simulink model "old"  (R2022b)
settings: Solver=FixedStepAuto  StartTime=1000  StopTime=1100  FixedStep=0.01  RelTol=1e-3
model workspace (MATLAB code in the model file):
  | A = ...
  |   [1 0.02;
  |    0 1];
  | 
  | B = [0.0002; 0.02];
  | 
  | C = [0 1];
  | 
  | I = ...
  |   [1 0;
  |    0 1];
  | 
  | P0 = ...
  |   [1 0;
  |    0 1];
  | 
  | PotenciaNegativa = -50000;
  | 
  | PotenciaPositiva = 80000;
  | 
  | Q = ...
  |   [10 0;
  |    0 10];
  | 
  | R = 1000;
  | 
  | T = 0.02;
  | 
  | TorqueMaxNegative = -12;
  | 
  | TorqueMaxPositive = 21;
  | 
  | diff_table_F = [0 0.0005 0.0005 0.0006 0.0006 0.0007 0.0008 0.0008 0.0009 ...
  |                 0.0009 0.001 0.0011 0.0011 0.0012 0.0013 0.0014 0.0014 ...
  |                 0.0015 0.0016 0.0017 0.0018 0.0018 0.0019 0.002 0.0021 ...
  |                 0.0022 0.0023 0.0024 0.0025 0.0026 0.0027 0.0027 0.0028 ...
  |                 0.0029 0.0031 0.0032 0.0033 0.0034 0.0035 0.0036 0.0037 ...
  |                 0.0038 0.0039 0.004 0.0042 0.0043 0.0044 0.0045 0.0046 ...
  |                 0.0048 0.0049 0.005 0.0051 0.0053 0.0054 0.0055 0.0057 ...
  |                 0.0058 0.0059 0.0061 0.0062 0.0064 0.0065 0.0067 0.0068 ...
  |                 0.007 0.0071 0.0073 0.0074 0.0076 0.0077 0.0079 0.008 0.0082 ...
  |                 0.0084 0.0085 0.0087 0.0089 0.009 0.0092 0.0094 0.0095];
  | 
  | diff_table_R = [0 0.0023 0.00253 0.00276 0.00299 0.00322 0.00345 0.00368 ...
  |                 0.00391 0.00414 0.00437 0.0046 0.00483 0.00506 0.00529 ...
  |                 0.00552 0.00575 0.00598 0.00621 0.00644 0.00667 0.0069 ...
  |                 0.00713 0.00736 0.00759 0.00782 0.00805 0.00828 0.00851 ...
  |                 0.00874 0.00897 0.0092 0.00943 0.00966 0.00989 0.01012 ...
  |                 0.01035 0.01058 0.01081 0.01104 0.01127 0.0115 0.01173 ...
  |                 0.01196 0.01219 0.01242 0.01265 0.01288 0.01311 0.01334 ...
  |                 0.01357 0.0138 0.01403 0.01426 0.01449 0.01472 0.01495 ...
  |                 0.01518 0.01541 0.01564 0.01587 0.0161 0.01633 0.01656 ...
  |                 0.01679 0.01702 0.01725 0.01748 0.01771 0.01794 0.01817 ...
  |                 0.0184 0.01863 0.01886 0.01909 0.01932 0.01955 0.01978 ...
  |                 0.02001 0.02024 0.02047 0.0207];
  | 
  | diff_table_ext_F = [0 0.0005 0.0005 0.0006 0.0006 0.0007 0.0008 0.0008 ...
  |                     0.0009 0.0009 0.001 0.0011 0.0011 0.0012 0.0013 0.0014 ...
  |                     0.0014 0.0015 0.0016 0.0017 0.0018 0.0018 0.0019 0.002 ...
  |                     0.0021 0.0022 0.0023 0.0024 0.0025 0.0026 0.0027 0.0027 ...
  |                     0.0028 0.0029 0.0031 0.0032 0.0033 0.0034 0.0035 0.0036 ...
  |                     0.0037 0.0038 0.0039 0.004 0.0042 0.0043 0.0044 0.0045 ...
  |                     0.0046 0.0048 0.0049 0.005 0.0051 0.0053 0.0054 0.0055 ...
  |                     0.0057 0.0058 0.0059 0.0061 0.0062 0.0064 0.0065 0.0067 ...
  |                     0.0068 0.007 0.0071 0.0073 0.0074 0.0076 0.0077 0.0079 ...
  |                     0.008 0.0082 0.0084 0.0085 0.0087 0.0089 0.009 0.0092 ...
  |                     0.0094 0.0095 0.0097 0.0099 0.01 0.0102 0.0104 0.0105 ...
  |                     0.0107 0.0109 0.011 0.0112 0.0114 0.0115 0.0117 0.0119 ...
  |                     0.012 0.0122 0.0124 0.0125 0.0127];
  | 
  | diff_table_ext_R = [0 0.0023 0.00253 0.00276 0.00299 0.00322 0.00345 0.00368 ...
  |                     0.00391 0.00414 0.00437 0.0046 0.00483 0.00506 0.00529 ...
  |                     0.00552 0.00575 0.00598 0.00621 0.00644 0.00667 0.0069 ...
  |                     0.00713 0.00736 0.00759 0.00782 0.00805 0.00828 0.00851 ...
  |                     0.00874 0.00897 0.0092 0.00943 0.00966 0.00989 0.01012 ...
  |                     0.01035 0.01058 0.01081 0.01104 0.01127 0.0115 0.01173 ...
  |                     0.01196 0.01219 0.01242 0.01265 0.01288 0.01311 0.01334 ...
  |                     0.01357 0.0138 0.01403 0.01426 0.01449 0.01472 0.01495 ...
  |                     0.01518 0.01541 0.01564 0.01587 0.0161 0.01633 0.01656 ...
  |                     0.01679 0.01702 0.01725 0.01748 0.01771 0.01794 0.01817 ...
  |                     0.0184 0.01863 0.01886 0.01909 0.01932 0.01955 0.01978 ...
  |                     0.02001 0.02024 0.02047 0.0207 0.02093 0.02116 0.02139 ...
  |                     0.02162 0.02185 0.02208 0.02231 0.02254 0.02277 0.023 ...
  |                     0.02323 0.02346 0.02369 0.02392 0.02415 0.02438 0.02461 ...
  |                     0.02484 0.02507];
  | 
  | pdl_threshold = 0.3;
  | 
  | r_torquedis = 0.7;
  | 
  | str_threshold = 1;
libraries: simulink_extras x5, dspfdesign x3, slpidlib x1
(part 2 of 2)

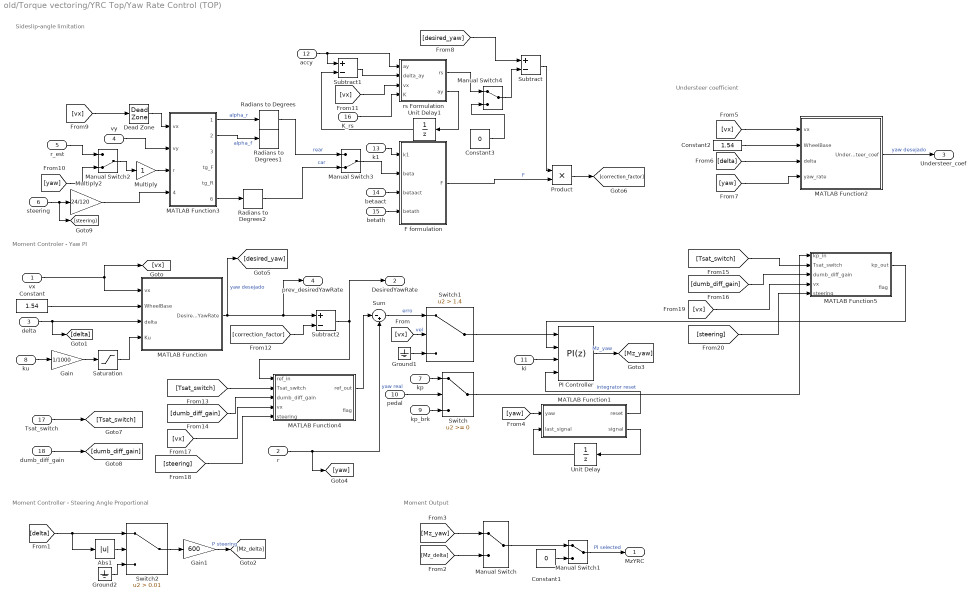
== system old/Torque vectoring/YRC Top/Yaw Rate Control (TOP) ==
  note: Sideslip-angle limitation
  note: Understeer coefficient
  note: Moment Controller - Steering Angle Proportional
  note: Moment Controler - Yaw PI
  note: Moment Output
  vx : Inport
  r : Inport  Port=2
  delta : Inport  Port=3
  vy : Inport  Port=4
  r_est : Inport  Port=5
  steering : Inport  Port=6
  kp : Inport  Port=7
  ku : Inport  Port=8
  kp_brk : Inport  Port=9
  pedal : Inport  Port=10
  ki : Inport  Port=11
  accy : Inport  Port=12
  k1 : Inport  Port=13
  betaact : Inport  Port=14
  betath : Inport  Port=15
  K_rs : Inport  Port=16
  Tsat_switch : Inport  Port=17
  dumb_diff_gain : Inport  Port=18
  Abs1 : Abs  SaturateOnIntegerOverflow=off
  Constant : Constant  Value=1.54
  Constant1 : Constant  Value=0
  Constant2 : Constant  Value=1.54
  Constant3 : Constant  Value=0
  Dead Zone : DeadZone
  F formulation : MATLAB Function  TreatAsAtomicUnit=on
  Gain : Gain  Gain=1/1000
  Gain1 : Gain  Gain=600
  Ground1 : Ground
  Ground2 : Ground
  MATLAB Function : MATLAB Function  TreatAsAtomicUnit=on
  MATLAB Function1 : MATLAB Function  TreatAsAtomicUnit=on
  MATLAB Function2 : MATLAB Function  TreatAsAtomicUnit=on
  MATLAB Function3 : MATLAB Function  TreatAsAtomicUnit=on
  MATLAB Function4 : MATLAB Function  TreatAsAtomicUnit=on
  MATLAB Function5 : MATLAB Function  TreatAsAtomicUnit=on
  Manual Switch : ManualSwitch
  Manual Switch1 : ManualSwitch
  Manual Switch2 : ManualSwitch  CurrentSetting=0
  Manual Switch3 : ManualSwitch  CurrentSetting=0
  Manual Switch4 : ManualSwitch
  Multiply : Gain
  Multiply2 : Gain  Gain=24/120
  PI Controller : slpidlib/PID Controller  Controller=PI  Form=Parallel  TimeDomain=Discrete-time  UseExternalTs=off  SampleTime=-1  IntegratorMethod=Backward Euler  FilterMethod=Forward Euler  ControllerParametersSource=external  P=400  I=100  UseKiTs=off  D=10  N=1  UseFilter=on  TunerSelectOption=Transfer Function Based (PID Tuner App)  InitialConditionSource=internal  InitialConditionForIntegrator=0  InitialConditionForFilter=0  DifferentiatorICPrevScaledInput=0  ExternalReset=rising  TrackingMode=off  Kt=1  LimitOutput=on  SatLimitsSource=internal  UpperSaturationLimit=1700  LowerSaturationLimit=-1700  LinearizeAsGain=off  AntiWindupMode=clamping  Kb=6  LimitIntegrator=off  UpperIntegratorSaturationLimit=inf  LowerIntegratorSaturationLimit=-inf  POutMin=[]  POutMax=[]  IOutMin=[]  IOutMax=[]  DOutMin=[]  DOutMax=[]  NOutMin=[]  NOutMax=[]  SumOutMin=[]  SumOutMax=[]  SaturationOutMin=[]  SaturationOutMax=[]  PParamMin=[]  PParamMax=[]  IParamMin=[]  IParamMax=[]  DParamMin=[]  DParamMax=[]  NParamMin=[]  NParamMax=[]  KbParamMin=[]  KbParamMax=[]  KtParamMin=[]  KtParamMax=[]  KbOutMin=[]  KbOutMax=[]  KtOutMin=[]  KtOutMax=[]  IntegratorOutMin=[]  IntegratorOutMax=[]  FilterOutMin=[]  FilterOutMax=[]  SumI1OutMin=[]  SumI1OutMax=[]  SumI2OutMin=[]  SumI2OutMax=[]  SumI3OutMin=[]  SumI3OutMax=[]  SumI4OutMin=[]  SumI4OutMax=[]  SumDOutMin=[]  SumDOutMax=[]  DifferentiatorOutMin=[]  DifferentiatorOutMax=[]  FilterDiffOutCoefMin=[]  FilterDiffOutCoefMax=[]  ReciprocalOutMin=[]  ReciprocalOutMax=[]  SumDenOutMin=[]  SumDenOutMax=[]  SumNumOutMin=[]  SumNumOutMax=[]  DivideOutMin=[]  DivideOutMax=[]  UdiffTsProdOutMin=[]  UdiffTsProdOutMax=[]  NTsProdOutMin=[]  NTsProdOutMax=[]  UintegralTsProdOutMin=[]  UintegralTsProdOutMax=[]  UngainTsProdOutMin=[]  UngainTsProdOutMax=[]  IntegratorContinuousStateAttributes=''  IntegratorStateMustResolveToSignalObject=off  IntegratorRTWStateStorageClass=Auto  FilterContinuousStateAttributes=''  FilterStateMustResolveToSignalObject=off  FilterRTWStateStorageClass=Auto  ParallelPVariant=ExternalParameters  IdealPVariant=Disabled  IVariant=ExternalParameters  DVariant=Disabled  IntegratorVariant=Discrete  SatVariant=Enabled  AWVariant=DiscClampingParallel  PCopyVariant=Disabled  TRVariant=Disabled  FdbkBlocksVariant=Feedback  IdealPFdbkVariant=Passthrough  SatFdbkVariant=Passthrough  DerivativeFilterVariant=Disabled  NVariant=Disabled  NCopyVariant=Disabled_SignalSpec  FilterICVariant=Disabled  IntegratorICVariant=InternalICs  ExternalResetVariant=ExternalReset  TRSumVariant=Passthrough  SumFdbkVariant=Enabled  SumVariant=Sum_PI  TsampFilterVariant=InternalTs  TsampNgainVariant=Passthrough  TsampIntegralVariant=Disabled_SignalSpec  ExternalSaturationOutDataTypeStr=Inherit: Same as second input
  Product : Product
  Radians to Degrees : simulink_extras/Transformations/Radians to Degrees
  Radians to Degrees1 : simulink_extras/Transformations/Radians to Degrees
  Radians to Degrees2 : simulink_extras/Transformations/Radians to Degrees
  Saturation : Saturate  UpperLimit=0.015  LowerLimit=0
  Subtract : Sum  Inputs=+-
  Subtract1 : Sum  Inputs=+-
  Subtract2 : Sum  Inputs=+-
  Sum : Sum  Inputs=|-+
  Switch : Switch  SaturateOnIntegerOverflow=off  InputSameDT=off
  Switch1 : Switch  Criteria=u2 > Threshold  Threshold=1.4  SaturateOnIntegerOverflow=off  InputSameDT=off
  Switch2 : Switch  Criteria=u2 > Threshold  Threshold=0.01  SaturateOnIntegerOverflow=off  InputSameDT=off
  Unit Delay : UnitDelay  SampleTime=-1  HasFrameUpgradeWarning=on
  Unit Delay1 : UnitDelay  SampleTime=-1  HasFrameUpgradeWarning=on
  rs Formulation : MATLAB Function  TreatAsAtomicUnit=on
  "MzYRC " : Outport  VectorParamsAs1DForOutWhenUnconnected=off
  DesiredYawRate : Outport  Port=2
  Understeer_coef : Outport  Port=3
  prev_desiredYawRate : Outport  Port=4
  wires:
  vx/1 -> MATLAB Function/1(vx), [vx]
  delta/1 -> MATLAB Function/3(delta), [delta]
  Sum/1 -> Switch1/1  "erro"
  r/1 -> [yaw], Sum/2  "yaw real"
  [delta] -> Abs1/1, Switch2/1
  Abs1/1 -> Switch2/2
  Switch2/1 -> Gain1/1
  Ground2/1 -> Switch2/3
  Manual Switch/1 -> Manual Switch1/1
  Manual Switch1/1 -> "MzYRC "/1  "PI selected"
  [vx] -> Switch1/2  "vel"
  Gain1/1 -> [Mz_delta]  "P steering"
  [Mz_delta] -> Manual Switch/2
  [Mz_yaw] -> Manual Switch/1
  Constant/1 -> MATLAB Function/2(WheelBase)
  MATLAB Function/1(DesiredYawRate) -> prev_desiredYawRate/1, Subtract2/1, [desired_yaw]  "yaw desejado"
  Ground1/1 -> Switch1/3
  Constant1/1 -> Manual Switch1/2
  PI Controller/1 -> [Mz_yaw]  "Mz_yaw"
  Switch1/1 -> PI Controller/1
  Gain/1 -> Saturation/1
  ku/1 -> Gain/1
  Saturation/1 -> MATLAB Function/4(Ku)
  pedal/1 -> Switch/2
  kp/1 -> Switch/1
  kp_brk/1 -> Switch/3
  ki/1 -> PI Controller/3
  MATLAB Function1/1(reset) -> PI Controller/4  "integrator reset"
  [yaw] -> MATLAB Function1/1(yaw)
  MATLAB Function1/2(signal) -> Unit Delay/1
  Unit Delay/1 -> MATLAB Function1/2(last_signal)
  MATLAB Function2/1(Understeer_coef) -> Understeer_coef/1  "yaw desejado"
  [vx] -> MATLAB Function2/1(vx)
  Constant2/1 -> MATLAB Function2/2(WheelBase)
  [delta] -> MATLAB Function2/3(delta)
  [yaw] -> MATLAB Function2/4(yaw_rate)
  vy/1 -> MATLAB Function3/2(vy)
  MATLAB Function3/1(alpha_r) -> Radians to Degrees/1  "alpha_r"
  MATLAB Function3/2(alpha_f) -> Radians to Degrees1/1  "alpha_f"
  [vx] -> Dead Zone/1
  r_est/1 -> Manual Switch2/1
  [yaw] -> Manual Switch2/2
  steering/1 -> [steering], Multiply2/1
  Multiply2/1 -> MATLAB Function3/4("steering ")
  Radians to Degrees/1 -> Manual Switch3/1  "rear"
  MATLAB Function3/6(alpha_car) -> Radians to Degrees2/1
  [desired_yaw] -> Subtract/1
  rs Formulation/1(rs) -> Manual Switch4/1
  Subtract/1 -> Product/1
  F formulation/1(F) -> Product/2  "F"
  Product/1 -> [correction_factor]
  [vx] -> rs Formulation/3(vx)
  rs Formulation/2(ay) -> Unit Delay1/1
  Unit Delay1/1 -> Subtract1/2
  accy/1 -> rs Formulation/1("ay "), Subtract1/1
  Subtract1/1 -> rs Formulation/2(delta_ay)
  Manual Switch3/1 -> F formulation/2(beta)
  Radians to Degrees2/1 -> Manual Switch3/2  "car"
  k1/1 -> F formulation/1(k1)
  betaact/1 -> F formulation/3(betaact)
  betath/1 -> F formulation/4(betath)
  Subtract2/1 -> MATLAB Function4/1(ref_in), DesiredYawRate/1
  [correction_factor] -> Subtract2/2
  Dead Zone/1 -> MATLAB Function3/1(vx)
  K_rs/1 -> rs Formulation/4(K)
  Multiply/1 -> MATLAB Function3/3(r)
  Manual Switch2/1 -> Multiply/1
  Manual Switch4/1 -> Subtract/2
  Constant3/1 -> Manual Switch4/2
  dumb_diff_gain/1 -> [dumb_diff_gain]
  Tsat_switch/1 -> [Tsat_switch]
  [Tsat_switch] -> MATLAB Function4/2(Tsat_switch)
  [dumb_diff_gain] -> MATLAB Function4/3(dumb_diff_gain)
  MATLAB Function4/1(ref_out) -> Sum/1
  Switch/1 -> MATLAB Function5/1(kp_in)
  [Tsat_switch] -> MATLAB Function5/2(Tsat_switch)
  [dumb_diff_gain] -> MATLAB Function5/3(dumb_diff_gain)
  MATLAB Function5/1(kp_out) -> PI Controller/2
  [vx] -> MATLAB Function4/4(vx)
  [steering] -> MATLAB Function4/5(steering)
  [vx] -> MATLAB Function5/4(vx)
  [steering] -> MATLAB Function5/5(steering)

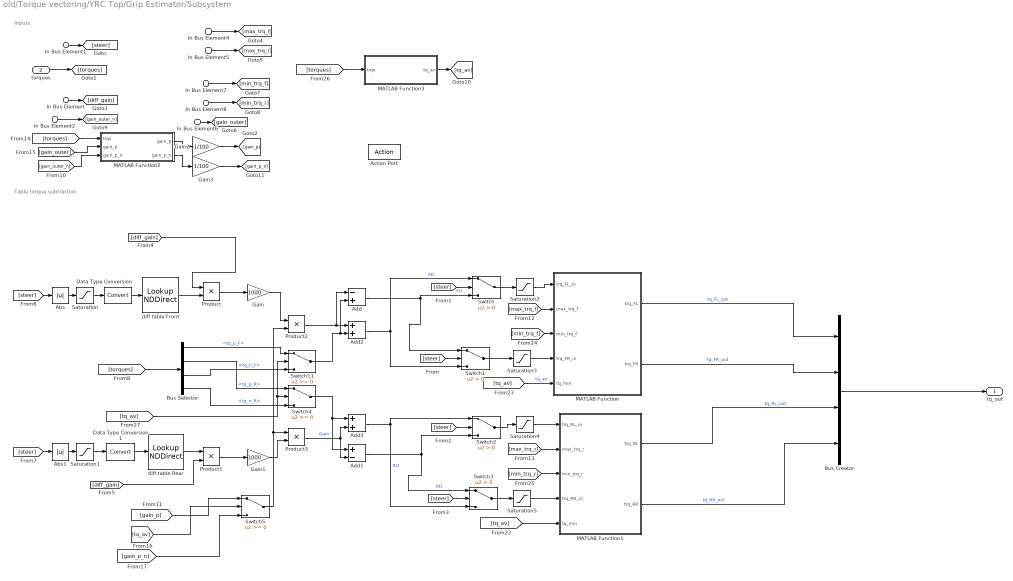
== system old/Torque vectoring/YRC Top/Grip Estimator/Subsystem ==
  note: Inputs
  note: Table torque subtraction
  In Bus Element1 : Inport  PortName=sensors  Element=steering
  torques : Inport  Port=2
  In Bus Element : Inport  Port=3  PortName=params  Element=diff_gain
  In Bus Element4 : Inport  Port=3  PortName=params  Element=max_trq_p_f
  In Bus Element5 : Inport  Port=3  PortName=params  Element=max_trq_p_r
  In Bus Element6 : Inport  Port=3  PortName=params  Element=gain_outer
  In Bus Element7 : Inport  Port=3  PortName=params  Element=max_trq_n_f
  In Bus Element8 : Inport  Port=3  PortName=params  Element=max_trq_n_r
  In Bus Element2 : Inport  Port=3  PortName=params  Element=gain_outer_n
  Action Port : ActionPort
  Abs : Abs  SaturateOnIntegerOverflow=off
  Abs1 : Abs  SaturateOnIntegerOverflow=off
  Add : Sum  Inputs=-+
  Add1 : Sum  Inputs=+-
  Add2 : Sum
  Add3 : Sum
  Bus Creator : BusCreator  Inputs=4
  Bus Selector : BusSelector  OutputSignals=tq_p_F,tq_p_R,tq_n_F,tq_n_R
  Data Type Conversion : DataTypeConversion  SaturateOnIntegerOverflow=off  RndMeth=Floor
  Data Type Conversion1 : DataTypeConversion  SaturateOnIntegerOverflow=off  RndMeth=Floor
  Gain : Gain  Gain=1000
  Gain1 : Gain  Gain=1000
  Gain2 : Gain  Gain=1/100
  Gain3 : Gain  Gain=1/100
  MATLAB Function : MATLAB Function  TreatAsAtomicUnit=on
  MATLAB Function1 : MATLAB Function  TreatAsAtomicUnit=on
  MATLAB Function2 : MATLAB Function  TreatAsAtomicUnit=on
  MATLAB Function3 : MATLAB Function  TreatAsAtomicUnit=on
  Product{,1..3} (4 alike) : Product
  Saturation : Saturate  UpperLimit=100  LowerLimit=0  ZeroCross=off
  Saturation1 : Saturate  UpperLimit=100  LowerLimit=0  ZeroCross=off
  Saturation{2..5} (4 alike) : Saturate  UpperLimit=21000  LowerLimit=-21000  ZeroCross=off
  Switch{,1..3} (4 alike) : Switch  Criteria=u2 > Threshold  SaturateOnIntegerOverflow=off  InputSameDT=off
  Switch11 : Switch  SaturateOnIntegerOverflow=off  InputSameDT=off
  Switch4 : Switch  SaturateOnIntegerOverflow=off  InputSameDT=off
  Switch5 : Switch  SaturateOnIntegerOverflow=off  InputSameDT=off
  diff table Front : LookupNDDirect  NumberOfTableDimensions=1  Table=diff_table_ext_F
  diff table Rear : LookupNDDirect  NumberOfTableDimensions=1  Table=diff_table_ext_R
  tq_out : Outport  VectorParamsAs1DForOutWhenUnconnected=off
  wires:
  [max_trq_r] -> MATLAB Function1/2(max_trq_r)
  [steer] -> Switch3/2
  [diff_gain] -> Product/1
  Switch2/1 -> Saturation4/1
  [steer] -> Switch2/2
  [steer] -> Abs1/1
  Gain/1 -> Product2/1
  In Bus Element1/1 -> [steer]
  Product1/1 -> Gain1/1
  [torques] -> Bus Selector/1
  Abs1/1 -> Saturation1/1
  Data Type Conversion/1 -> diff table Front/1
  Add2/1 -> Switch1/3, Switch/1  "FD"
  MATLAB Function1/1(trq_RL) -> Bus Creator/3  "tq_RL_out"
  In Bus Element8/1 -> [min_trq_r]
  In Bus Element6/1 -> [gain_outer]
  [gain_outer] -> MATLAB Function2/2("gain_p ")
  [max_trq_f] -> MATLAB Function/2(max_trq_f)
  MATLAB Function2/1(gain_p) -> Gain2/1
  Saturation5/1 -> MATLAB Function1/4(trq_RR_in)
  [torques] -> MATLAB Function2/1(trqs)
  In Bus Element5/1 -> [max_trq_r]
  Bus Selector/2 -> Switch4/1  "<tq_p_R>"
  Bus Creator/1 -> tq_out/1
  [tq_av] -> MATLAB Function1/5(tq_min)
  Gain1/1 -> Product3/2
  [min_trq_f] -> MATLAB Function/3(min_trq_f)
  [diff_gain] -> Product1/2
  [min_trq_r] -> MATLAB Function1/3(min_trq_r)
  [torques] -> MATLAB Function3/1(trqs)
  MATLAB Function3/1(tq_av) -> [tq_av]
  MATLAB Function2/2(gain_p_n) -> Gain3/1
  [steer] -> Switch/2
  torques/1 -> [torques]
  Switch11/1 -> Add/2, Add2/2
  In Bus Element/1 -> [diff_gain]
  [gain_outer_n] -> MATLAB Function2/3("gain_p_n ")
  Gain3/1 -> [gain_p_n]
  MATLAB Function/1(trq_FL) -> Bus Creator/1  "tq_FL_out"
  [tq_av] -> Switch5/2
  Switch/1 -> Saturation2/1
  diff table Rear/1 -> Product1/1
  In Bus Element2/1 -> [gain_outer_n]
  Saturation1/1 -> Data Type Conversion1/1
  Product/1 -> Gain/1
  [gain_p] -> Switch5/1
  Product3/1 -> Add1/2, Add3/2  "Gain"
  diff table Front/1 -> Product/2
  Saturation2/1 -> MATLAB Function/1(trq_FL_in)
  Bus Selector/4 -> Switch4/3  "<tq_n_R>"
  Switch3/1 -> Saturation5/1
  [tq_av] -> Switch11/2, Switch4/2
  Add3/1 -> Switch3/3, Switch2/1  "RU"
  Gain2/1 -> [gain_p]
  Bus Selector/3 -> Switch11/3  "<tq_n_F>"
  Saturation/1 -> Data Type Conversion/1
  Add1/1 -> Switch2/3, Switch3/1  "RD"
  Product2/1 -> Add2/1, Add/1
  Switch1/1 -> Saturation3/1
  In Bus Element7/1 -> [min_trq_f]
  Abs/1 -> Saturation/1
  [steer] -> Abs/1
  In Bus Element4/1 -> [max_trq_f]
  [steer] -> Switch1/2
  Switch4/1 -> Add1/1, Add3/1
  Switch5/1 -> Product2/2, Product3/1
  Add/1 -> Switch1/1, Switch/3  "FU"
  Saturation3/1 -> MATLAB Function/4(trq_FR_in)
  Bus Selector/1 -> Switch11/1  "<tq_p_F>"
  [tq_av] -> MATLAB Function/5(tq_min)  "tq_av"
  MATLAB Function1/2(trq_RR) -> Bus Creator/4  "tq_RR_out"
  MATLAB Function/2(trq_FR) -> Bus Creator/2  "tq_FR_out"
  Saturation4/1 -> MATLAB Function1/1(trq_RL_in)
  [gain_p_n] -> Switch5/3
  Data Type Conversion1/1 -> diff table Rear/1

== matlab function old/MATLAB Function3 ==
  data: torques_in input; torques_out output; trac_mode input
function torques_out  = check_trac(torques_in,trac_mode)

torques_out = torques_in;

if trac_mode == 1
    torques_out([1 2]) = 0;
elseif trac_mode == 2
    torques_out([3 4]) = 0;
end

== matlab function old/Torque vectoring/YRC Top/MATLAB Function ==
  data: steering input; delta_in input; x output; pedal input; omegas input; Mz_desired input; Tmax input; Tmin input; Pmax input; Pmin input; Regen_on_Acc input; Tsat input; error output; T_total output; exitflag output; diff_gain input
 function [x, error, T_total, exitflag] = TorqueDist(steering, delta_in, pedal,...
    omegas, Mz_desired, Tmax, Tmin, Pmax, Pmin, Regen_on_Acc, Tsat, diff_gain)

% Just for versioning Control
[x,error,T_total,exitflag] = QP_TorqueDist(steering,delta_in,pedal,omegas,...
    Mz_desired,Tmax,Tmin,Pmax,Pmin,Regen_on_Acc,Tsat,diff_gain);

== matlab function old/Torque vectoring/Differential Jardado/MATLAB Function1 ==
  data: trq_RL_in input; trq_RL output; max_trq_r input; min_trq_r input; trq_RR_in input; trq_RR output; tq_min input
function [trq_RL,trq_RR] = sat(trq_RL_in,max_trq_r,min_trq_r,trq_RR_in,tq_min)
    

    if tq_min<0
        trq_RL = max(trq_RL_in,-min_trq_r);
        trq_RR = max(trq_RR_in,-min_trq_r);       
    else
        trq_RL = min(trq_RL_in,max_trq_r);
        trq_RR = min(trq_RR_in,max_trq_r);
    end
    
    if trq_RL ~= trq_RL_in
       diff=trq_RL_in-trq_RR_in;
       trq_RR=trq_RL-diff;
    elseif trq_RR ~= trq_RR_in
        diff=trq_RR_in - trq_RL_in;
        trq_RL=trq_RR_in -diff;
    end
end

== matlab function old/Torque vectoring/YRC Top/Yaw Rate Control (TOP)/MATLAB Function1 ==
  data: yaw input; last_signal input; reset output; signal output
function [reset,signal] = Ireset(yaw,last_signal)

if sign(last_signal) ~= sign(yaw)
    reset = 1;
else
    reset = 0;
end
signal = sign(yaw);
end

== matlab function old/Torque vectoring/YRC Top/Yaw Rate Control (TOP)/MATLAB Function ==
  data: vx input; WheelBase input; DesiredYawRate output; delta input; Ku input
function DesiredYawRate  = YawRateCalc(vx, WheelBase, delta,Ku)
%#codegen
wb = WheelBase;
DesiredYawRate = (vx * tan(delta)) /(wb+Ku*vx^2);

== matlab function old/Torque vectoring/Differential Jardado/MATLAB Function2 ==
  data: trqs input; gain_p output; gain_p input; gain_p_n input; gain_p_n output
function [gain_p,gain_p_n] = fix_tomas(trqs, gain_p,gain_p_n)

% Tomas was dumb and made de walk move forward without APPS
if sum(trqs)==0
    gain_p = 0;
    gain_p_n=0;
end

== matlab function old/Torque vectoring/Differential Jardado/MATLAB Function3 ==
  data: trqs input; tq_av output
function tq_av= max_torque(trqs)

    trqs=trqs.*1000;
    tq_av=sum(trqs)/4;

== matlab function old/Pedal Proportional & Regen/Acc convertion ==
  data: brk_pedal input; acc_bias input; trq_p_F output; max_trq input; trq_p_R output; max_trq_F output; max_trq_R output
function [trq_p_F, trq_p_R,max_trq_F,max_trq_R] = acc_torque(brk_pedal,acc_bias,max_trq)

    %% Calculate max torque for each axle
    %Break bias over 50% more torque in front axle
    if acc_bias>0.50
        max_trq_F=max_trq;
        max_trq_R=(max_trq*(1-acc_bias))/acc_bias;
    else
        max_trq_R=max_trq;
        max_trq_F=(max_trq*acc_bias)/(1-acc_bias);  
    end
    
    %% Calculate acc torque for Front Axle
    
    if brk_pedal>0.01
        trq_p_F = max_trq_F * brk_pedal;
    else
        trq_p_F = 0;
    end
    
    %% Calculate acc torque for Front Axle
    if brk_pedal>0.01
        trq_p_R = max_trq_R * brk_pedal;
    else
        trq_p_R = 0;
    end
end

== matlab function old/Torque vectoring/YRC Top/Yaw Rate Control (TOP)/MATLAB Function2 ==
  data: vx input; WheelBase input; Understeer_coef output; delta input; yaw_rate input
function Understeer_coef  = YawRateCalc(vx, WheelBase, delta,yaw_rate)
%#codegen
wb = WheelBase;
Understeer_coef = (((vx * tan(delta))/yaw_rate)-wb) /(vx^2);

== matlab function old/Torque vectoring/YRC Top/Grip Estimator/Subsystem/MATLAB Function ==
  data: trq_FL_in input; trq_FL output; max_trq_f input; min_trq_f input; trq_FR_in input; trq_FR output; tq_min input
function [trq_FL,trq_FR] = sat(trq_FL_in,max_trq_f,min_trq_f,trq_FR_in,tq_min)
    
    

    if tq_min<0
        trq_FL = max(trq_FL_in,-min_trq_f);
        trq_FR = max(trq_FR_in,-min_trq_f);       
    else
        trq_FL = min(trq_FL_in,max_trq_f);
        trq_FR = min(trq_FR_in,max_trq_f);
    end

    if trq_FL ~= trq_FL_in
       diff=trq_FL_in-trq_FR_in;
       trq_FR=trq_FL-diff;
    elseif trq_FR ~= trq_FR_in
        diff=trq_FR_in - trq_FL_in;
        trq_FL=trq_FR_in -diff;
    end
    
end

== matlab function old/Torque vectoring/YRC Top/Grip Estimator/Subsystem/MATLAB Function1 ==
  data: trq_RL_in input; trq_RL output; max_trq_r input; min_trq_r input; trq_RR_in input; trq_RR output; tq_min input
function [trq_RL,trq_RR] = sat(trq_RL_in,max_trq_r,min_trq_r,trq_RR_in,tq_min)
    

    if tq_min<0
        trq_RL = max(trq_RL_in,-min_trq_r);
        trq_RR = max(trq_RR_in,-min_trq_r);       
    else
        trq_RL = min(trq_RL_in,max_trq_r);
        trq_RR = min(trq_RR_in,max_trq_r);
    end
    
    if trq_RL ~= trq_RL_in
       diff=trq_RL_in-trq_RR_in;
       trq_RR=trq_RL-diff;
    elseif trq_RR ~= trq_RR_in
        diff=trq_RR_in - trq_RL_in;
        trq_RL=trq_RR_in -diff;
    end
end

== matlab function old/Torque vectoring/YRC Top/Grip Estimator/Subsystem/MATLAB Function2 ==
  data: trqs input; gain_p output; gain_p input; gain_p_n input; gain_p_n output
function [gain_p,gain_p_n] = fix_tomas(trqs, gain_p,gain_p_n)

% Tomas was dumb and made de walk move forward without APPS
if sum(trqs)==0
    gain_p = 0;
    gain_p_n=0;
end

== matlab function old/Torque vectoring/YRC Top/Grip Estimator/Subsystem/MATLAB Function3 ==
  data: trqs input; tq_av output
function tq_av= max_torque(trqs)

    trqs=trqs.*1000;
    tq_av=sum(trqs)/4;

== matlab function old/Torque vectoring/YRC Top/Yaw Rate Control (TOP)/MATLAB Function3 ==
  data: vx input; alpha_r output; vy input; r input; steering input; alpha_f output; steering output; tg_F output; tg_R output; alpha_car output
function [alpha_r,alpha_f,steering,tg_F,tg_R,alpha_car] = fcn(vx, vy, r, steering)

    l_f=0.72;
    l_r=0.82;
    
    alpha_f = (steering*2*pi)/360 - atan2(vy + r*l_f, vx);
    alpha_r = atan2((vy - r*l_r), vx);
    
    steering=(steering*2*pi)/360;
    
    tg_F=atan2(vy + r*l_f, vx);
    tg_R=atan2((vy - r*l_r), vx);
    
    alpha_car=atan2(vy,vx);
    
    if vx<4
        alpha_r=0;
        alpha_f=0;
        alpha_car=0;
    end

== matlab function old/Torque vectoring/YRC Top/Yaw Rate Control (TOP)/F formulation ==
  data: k1 input; F output; beta input; betaact input; betath input
function F = fcn(k1,beta,betaact,betath)

    F=0;

    if abs(beta)<betaact
        
        F=0;
        
    elseif abs(beta)>betath
        
        F=k1;
        
    elseif abs(beta)>betaact
        
        F=k1*(abs(beta)-betaact)/(betath-betaact);
        
    end

== matlab function old/Torque vectoring/YRC Top/Yaw Rate Control (TOP)/rs Formulation ==
  data: ay input; rs output; delta_ay input; vx input; ay output; K input
function [rs,ay] = fcn(ay,delta_ay,vx,K)
    
    if abs(ay)<delta_ay
        
        rs=0;
        
    else
        
        rs=(ay-K*sign(ay)*delta_ay)/vx;
        
    end

    if vx<3
        
        rs=0;
        
    end
    
    % To erase this component in the code when testing if necessary
    if (K*10)==127
        rs=0;
    end

== matlab function old/Torque vectoring/Switch Case Action Subsystem1/MATLAB Function ==
  data: APPS input; BPPS input; steer input; Ax input; vx input; max_tq_f input; tq_FL_out output; tq_FR_out output; tq_RL_out output; tq_RR_out output; max_tq_r input; min_tq_f input; min_tq_r input; diff_gain input; diff output; ratio output
function [tq_FL_out, tq_FR_out, tq_RL_out, tq_RR_out, diff, ratio] = fcn(APPS, BPPS, steer, Ax, vx, max_tq_f, max_tq_r, min_tq_f, min_tq_r, diff_gain)

diff = (0.0221*power(steer, 3) - 1.83*steer*vx - 0.6574*steer) * diff_gain;

ratio = max(min(Ax/9.81,1), -1)*0.16;

if BPPS > 0
    tq_FL_out = (min_tq_f*BPPS + diff/2*(0.4-ratio));
    tq_FR_out = (min_tq_f*BPPS - diff/2*(0.4-ratio));
    tq_RL_out = (min_tq_r*BPPS + diff/2*(0.6+ratio));
    tq_RR_out = (min_tq_r*BPPS - diff/2*(0.6+ratio));
elseif APPS > 0
    tq_FL_out = (max_tq_f*APPS + diff/2*(0.4-ratio));
    tq_FR_out = (max_tq_f*APPS - diff/2*(0.4-ratio));
    tq_RL_out = (max_tq_r*APPS + diff/2*(0.6+ratio));
    tq_RR_out = (max_tq_r*APPS - diff/2*(0.6+ratio));
else 
    tq_FL_out = 0;
    tq_FR_out = 0;
    tq_RL_out = 0;
    tq_RR_out = 0;
end

tq = [tq_FL_out, tq_FR_out, tq_RL_out, tq_RR_out];
for i = 1:size(tq,2)
    if tq(i) > 21
        tq(i) = 21;
    elseif tq(i) < -21
        tq(i) = -21;
    end
    tq(i) = tq(i)*1000;
end

tq_FL_out = tq(1);
tq_FR_out = tq(2);
tq_RL_out = tq(3);
tq_RR_out = tq(4);

== matlab function old/Torque vectoring/Differential Jardado/MATLAB Function ==
  data: trq_FL_in input; trq_FL output; max_trq_f input; min_trq_f input; trq_FR_in input; trq_FR output; tq_min input
function [trq_FL,trq_FR] = sat(trq_FL_in,max_trq_f,min_trq_f,trq_FR_in,tq_min)
    
    

    if tq_min<0
        trq_FL = max(trq_FL_in,-min_trq_f);
        trq_FR = max(trq_FR_in,-min_trq_f);       
    else
        trq_FL = min(trq_FL_in,max_trq_f);
        trq_FR = min(trq_FR_in,max_trq_f);
    end

    if trq_FL ~= trq_FL_in
       diff=trq_FL_in-trq_FR_in;
       trq_FR=trq_FL-diff;
    elseif trq_FR ~= trq_FR_in
        diff=trq_FR_in - trq_FL_in;
        trq_FL=trq_FR_in -diff;
    end
    
end

== matlab function old/Torque vectoring/YRC Top/Yaw Rate Control (TOP)/MATLAB Function4 ==
  data: ref_in input; ref_out output; Tsat_switch input; dumb_diff_gain input; vx input; steering input; flag output
function [ref_out, flag] = fcn(ref_in, Tsat_switch, dumb_diff_gain, vx, steering)

if (Tsat_switch == 0 || Tsat_switch == 2) && vx < 3 && abs(steering) > 90
    ref_out = ref_in * (dumb_diff_gain / 10);
    flag = 1;
else
    ref_out = ref_in;
    flag = 0;
end

== matlab function old/Torque vectoring/YRC Top/Yaw Rate Control (TOP)/MATLAB Function5 ==
  data: kp_in input; kp_out output; Tsat_switch input; dumb_diff_gain input; vx input; steering input; flag output
function [kp_out, flag] = fcn(kp_in, Tsat_switch, dumb_diff_gain, vx, steering)

if (Tsat_switch == 1 || Tsat_switch == 2) && vx < 3 && abs(steering) > 90
    kp_out = kp_in * (dumb_diff_gain / 10);
    flag = 1;
else
    kp_out = kp_in;
    flag = 0;
end

== matlab function old/Pedal Proportional & Regen/MATLAB Function ==
  data: brk_pedal input; regen_bias input; trq_n_F output; min_trq input; trq_n_R output; min_trq_R output; min_trq_F output
function [trq_n_F, trq_n_R,min_trq_R,min_trq_F] = regen_torque(brk_pedal,regen_bias,min_trq)

    %% Calculate max torque for each axle
    %Break bias over 50% more torque in front axle
    if regen_bias>0.50
        min_trq_F=min_trq;
        min_trq_R=(min_trq*(1-regen_bias))/regen_bias;
    else
        min_trq_R=min_trq;
        min_trq_F=(min_trq*regen_bias)/(1-regen_bias);  
    end
    
    %% Calculate regen torque for Front Axle
    
    if brk_pedal<-0.01
        trq_n_F = min_trq_F * brk_pedal;
    else
        trq_n_F = 0;
    end
    
    %% Calculate regen torque for Front Axle
    
    if brk_pedal<-0.01
        trq_n_R = min_trq_R * brk_pedal;
    else
        trq_n_R = 0;
    end
    
end

== matlab function old/Torque vectoring/YRC Top/Grip Estimator/MATLAB Function2 ==
  data: Ax input; Tsat output; Ay input; v input; grip input; ARW1 output; ARW2 output; ARW3 output; ARW4 output; frontLatLT output; rearLatLT output; F_Ay_gain input; Ax_gain input; R_Ay_gain input; Aero_gain input
function [Tsat,ARW1,ARW2, ARW3,ARW4,frontLatLT,rearLatLT]  = fcn(Ax,Ay,v,grip, F_Ay_gain, Ax_gain, R_Ay_gain,Aero_gain)

    %% Car Parameters
    mass = 302; %Car weight + Pilot
    wb = 1.54; %wheelbase
    tf = 1.2; tr = 1.2; %front and rear track
    hcg = 0.331; %height of the center of gravity
    weightDist = 0.48; %front weight distribuition
    FRS = 474; RRS = 380; %roll stiffness
    frontRCh = 0.039; %height of front roll center
    rearRCh = 0.060; %height of rear roll center height
    g = 9.81;
    Area = 1;
    CL = 4.64; %lift coefficient
    CD = 1.78; %drag coefficient
    ro = 1.23; 
    aero_dist = 0.48; %front aerodynamic distribuition
    a = 0.72; %longitudinal distance from front axle until CG
    b = 0.82; %longitudinal distance from CG until rear axle
    r = 0.235; %wheel radius
    GR = 15.21; %gear ratio
    mu_x = grip /100;
    S_mu = 0.00035;
    CRM = 0;
    
    %% Rest
    Tsat = zeros(4,1);
    [Fz1,Fz2,Fz3,Fz4,ARW1,ARW2,ARW3,ARW4,frontLatLT,rearLatLT]=load_distribution(mass,Ax,Ay,...
        wb,tf,tr,hcg,weightDist,1-weightDist,...
        FRS,RRS,frontRCh,rearRCh,g,Area,v,CL,ro,aero_dist,CRM,a,b,Ax_gain,F_Ay_gain,R_Ay_gain,Aero_gain);
    
    Fz1 = max(Fz1,100);
    Fz2 = max(Fz2,100);
    Fz3 = max(Fz3,100);
    Fz4 = max(Fz4,100);
    
    Tsat(1) = (Fz1 * max(mu_x - S_mu*Fz1, 1))/GR*r;
    Tsat(2) = (Fz2 * max(mu_x - S_mu*Fz2, 1))/GR*r;
    Tsat(3) = (Fz3 * max(mu_x - S_mu*Fz3, 1))/GR*r;
    Tsat(4) = (Fz4 * max(mu_x - S_mu*Fz4, 1))/GR*r;
    
end

function [Fz1,Fz2,Fz3,Fz4,ARW1,ARW2,ARW3,ARW4,frontLatLT,rearLatLT]=load_distribution(mass,Ax,Ay,...
        wheelbase,tf,tr,hcg,weightDistFront,weightDistRear,...
        FRS,RRS,frontRCHeight,rearRCHeight,g,Area,v,CL,ro,aero_dist,CRM,a,b,Ax_gain,F_Ay_gain,R_Ay_gain,Aero_gain)
    
    %% Initial calculations
    %RollAxisSlope=(rearRCHeight -frontRCHeight)/wheelbase;
    %RollAxisUnderCG=frontRCHeight + RollAxisSlope*a;
    %H=hcg - RollAxisUnderCG;
    
    
    %% Stacionary Load Distribution
    load_rear=weightDistRear*mass*g; %total force in the rear axle
    load_front=weightDistFront*mass*g; %total force in the front axle
    
    %% Front Lateral Transfer
    %frontLatLT=mass/tf*(H*FRS/(FRS+RRS)+b/wheelbase*frontRCHeight)*Ay;
    frontLatLT = ((mass*hcg*Ay)/tf)/2; 
    
    %% Rear Lateral Transfer
    %rearLatLT=mass/tr*(H*RRS/(FRS+RRS)+a/wheelbase*rearRCHeight)*Ay;
    rearLatLT = ((mass*hcg*Ay)/tr)/2;
    
    %% Longitudinal Weight transfer
    longLT=(mass*hcg*Ax)/wheelbase;
    
    %% Aerodinamic contribution
    %Front and rear Lift coefficient calculation
    CLfront=CL*aero_dist;
    CLrear=CL-CLfront;
    LF=CLfront*0.5*ro*(v^2)*Area;
    LR=CLrear*0.5*ro*(v^2)*Area;
    
    %load transfer duo to aerodynamic forces in each wheel
    ARW1= (-LF/2);
    ARW2= (-LF/2);
    ARW3= (-LR/2);
    ARW4= (-LR/2);
    
    
    %% Total Fz in each Wheel
    Fz1 = load_front/2 - Ax_gain*longLT/2 - F_Ay_gain*frontLatLT - Aero_gain*ARW1;
    Fz2 = load_front/2 - Ax_gain*longLT/2 + F_Ay_gain*frontLatLT - Aero_gain*ARW2;
    Fz3 = load_rear/2  + Ax_gain*longLT/2 - R_Ay_gain*rearLatLT  - Aero_gain*ARW3;
    Fz4 = load_rear/2  + Ax_gain*longLT/2 + R_Ay_gain*rearLatLT  - Aero_gain*ARW4;

end

== matlab function old/Torque vectoring/YRC Top/MATLAB Function2 ==
  data: pedal input; trq output; trq input
function trq = safety(pedal,trq)


    if pedal == 0
        trq = trq.*0;
    end
    
    if pedal < 0
        trq = min(0,trq);
    end
end

== matlab function old/Torque vectoring/YRC Top/Alternavie Regen algorithms/MATLAB Function2 ==
  data: min_trq input; trq output; Tsat input
function trq = regen_limits(min_trq,Tsat)
    trq = zeros(4,1);
    
    for i=1:4
        trq(i) = min(min_trq(i),Tsat(i));
    end
end

== matlab function old/Torque vectoring/YRC Top/MATLAB Function3 ==
  data: Tmax_in input; Tmax_out output; trac_mode input
function Tmax_out  = check_trac(Tmax_in,trac_mode)

Tmax_out = Tmax_in;

if trac_mode == 1
    Tmax_out([1 2]) = 0;
elseif trac_mode == 2
    Tmax_out([3 4]) = 0;
end

== matlab function old/Torque vectoring/YRC Top/MATLAB Function4 ==
  data: Tmin_in input; Tmin_out output; trac_mode input
function Tmin_out  = check_trac(Tmin_in,trac_mode)

Tmin_out = Tmin_in;

if trac_mode == 1
    Tmin_out([1 2]) = 0;
elseif trac_mode == 2
    Tmin_out([3 4]) = 0;
end
